simulink model "Flexible_Beam_LP_Simple"  (R2014a)
settings: Solver=ode23t  StartTime=0.0  StopTime=200  RelTol=1e-3  AbsTol=1e-6
PreLoadFcn:
  | Cantilever_Beam_MS2G_Parameters
PostLoadFcn:
  | warning off Simulink:Engine:UsingDefaultMaxStepSize
  | warning off Simulink:Engine:SaveWithParameterizedLinks_Warning
undefined symbols (not defined in the file or in its folder): beam_wall, beam_width, Extr_Data_Box, X, Y, Z
undefined symbols (not defined in the file): beam_length, Damping, density, kbendingx, kbendingy, kelongz, ktwistz, num_elem, shearM, youngsM
libraries: sm_lib x217, nesl_utility x5
(part 1 of 6)
Description:
  | Copyright 2014 The MathWorks, Inc.
settings Model: Creator=smiller  LastModifiedBy=smiller
settings DebuggingCC: UnderspecifiedInitializationDetection=Classic  StateNameClashWarn=warning
settings ExplorerConfigSet: InternalSimMechanicsExplorerSettings="<ExplorerConfiguration><canonicalview>default</canonicalview><AnimationSetting><BasePlaybackSpeed>1.0</BasePlaybackSpeed><PlaybackSpeedFactor>1.0</PlaybackSpeedFactor></AnimationSetting><TilePanel><TileInfo><Tiles Columns=\"1\" Count=\"1\" Rows=\"1\"><Column Left=\"2\" Weight=\"1\"/><Column Left=\"626\"/><Row Top=\"2\" Weight=\"1\"/><Row Top=\"393\"/><Tile Height=\"1\" Width=\"1\" X=\"0\" Y=\"0\"/></Tiles></TileInfo><SceneInfo><SceneViewer><BGColor><R>0.60000002384185791</R><G>0.60000002384185791</G><B>0.60000002384185791</B></BGColor><Camera><Position><X>46.577974053951756</X><Y>-0.39590861008534267</Y><Z>0.29453050072829112</Z></Position><Center><X>15.001379163844208</X><Y>-0.52106864873913594</Y><Z>0.1428630073847893</Z></Center><Up><X>-0.0040091656961971532</X><Y>0.99994673738277207</Y><Z>0.0095104672845314226</Z></Up><Left>-1.0637916226228141</Left><Right>1.0637916226228141</Right><Bottom>-1.031964585942253</Bottom><Top>1.031964585942253</Top></Camera></SceneViewer></SceneInfo></TilePanel></ExplorerConfiguration>"

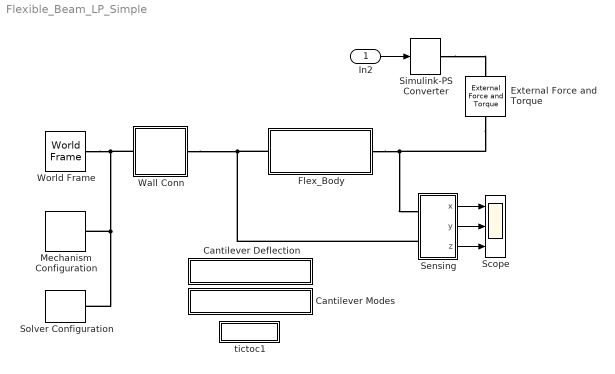
== system Flexible_Beam_LP_Simple ==
  In2 : Inport
  Cantilever Deflection : Subsystem
      settings: OpenFcn=|
      | mdl = bdroot;
      | 
      | load_system('FlexBeamElement_MS2G_Lib')
      | set_param('FlexBeamElement_MS2G_Lib', 'Lock', 'off');
      | set_param('FlexBeamElement_MS2G_Lib/Flex_Element','BlockChoice','Full')
      | 
      | open_system(mdl);
      | open_system([mdl, '/Scope']);
      | set_param([bdroot '/Wall Conn'],'OverrideUsingVariant','Fixed');
      | %set_param([mdl, '/Sensing/Transform Sensor'],'MeasurementFrame','World')
      | 
      | sim(mdl);
      | disp(['Static Deflection is ' num2str(TipDef.signals(2).values(end)) ' m'])
      mask Display: disp('Cantilever Deflection');
  Cantilever Modes : Subsystem
      settings: OpenFcn=Cantilever_Modes_Shapes_MS2G
      mask Display: disp('Cantilever Modes');
  External Force and Torque : sm_lib/Forces and Torques/External Force and Torque  ForceResolutionFrame=AttachedFrame  EnableForceX=off  EnableForceY=on  EnableForceZ=off  EnableForce=off  TorqueResolutionFrame=AttachedFrame  EnableTorqueX=off  EnableTorqueY=off  EnableTorqueZ=off  EnableTorque=off  BlockFunction=simmechanics.library.forces_torques.external_force_torque
  Flex_Body : Subsystem  mask(Flexible Body){rho=density, youngsM=youngsM, shearM=shearM, numelem=num_elem, beam_length=beam_length, beam_width=beam_width, beam_wall=beam_wall, b=Damping}
      mask prompts: rho "Material Density (kg/(m^3)"; youngsM "Modulus of Elasticity (N/m2)"; shearM "Shear Modulus (N/m2)"; numelem "Number of elements"; beam_length "Beam Length (m)"; beam_width "Beam Width & Height (m)"; beam_wall "Beam Wall Thickness(m)"; b "Damping Constant (Nm/rad.s)"
      mask help:
      | Models a flexible hollow square beam based on lumped parameter method.
      | Number of flexible elements, material properties as well as beam
      | dimension can be varied from mask parameters.
      mask init:
      | [kbendingx, kbendingy, ktwistz, kelongz, length] = Compute_GFE_Prop(rho, youngsM, shearM, numelem, beam_length, beam_width,beam_wall);
      | thisblock = gcb;
      | anno = ['No of Elem: ' num2str(numelem)];
      | set_param(thisblock, 'AttributesFormatString',anno);
      | if numelem <1
      |     error('Number of Flexible elements should be greater than 0')
      | end
      | prev_flex_bod = find_system(gcb,'LookUnderMasks','all','RegExp','on','Name','Flex_Elem_*');
      | if ~isempty(prev_flex_bod)
      |     delete_block(prev_flex_bod(1:end))
      | end
      | linehan = find_system(thisblock,'LookUnderMasks','all','FindAll','on','type','line');
      | if ~isempty(linehan)
      |     delete_line(linehan)
      | end
      | blk_or = [100 155 140 195];
      | set_param([thisblock '/B'],'Position',blk_or)
      | set_param([thisblock '/' sprintf('Transform\nBeamX')],'Position',blk_or+[80 0 80 0])
      | add_line(thisblock,['B/Rconn1'],[sprintf('Transform\nBeamX') '/Lconn1'],'autorouting','on');
      | add_block('FlexBeamElement_MS2G_Lib/Bend_Simple',[thisblock '/Flex_Elem_' num2str(1)],'Position',blk_or+[80 0 80 0]*2)
      | add_line(thisblock,[sprintf('Transform\nBeamX') '/Rconn1'],['Flex_Elem_' num2str(1) '/Lconn1'],'autorouting','on');
      | set_param([thisblock '/Flex_Elem_' num2str(1)], 'LinkStatus', 'none')
      | state_order{1} = [thisblock '/Flex_Elem_' num2str(1) '/Revolute Joint'];
      | for i = 2:1:numelem
      |     add_block('FlexBeamElement_MS2G_Lib/Bend_Simple',[thisblock '/Flex_Elem_' num2str(i)],'Position',blk_or+(i+1)*[80 0 80 0])
      |     add_line(thisblock,['Flex_Elem_' num2str(i-1) '/Rconn1'],['Flex_Elem_' num2str(i) '/Lconn1'],'autorouting','on');
      |     set_param([thisblock '/Flex_Elem_' num2str(i)], 'LinkStatus', 'none')
      |     state_order{i} = [thisblock '/Flex_Elem_' num2str(i) '/Revolute Joint'];
      | end
      | set_param([thisblock '/F'],'Position',blk_or+ (numelem+2)*[80 0 80 0]);
      | add_line(thisblock,['Flex_Elem_' num2str(numelem) '/Rconn1'],['F/Rconn1'],'autorouting','on');
      | assignin('base','State_order',state_order)
      settings: AttributesFormatString=No of Elem: 30  CopyFcn=set_param(gcb, 'LinkStatus', 'none')
      mask Display:
      | image(imread('Flexible_Beam.png'));
      | color red
      | port_label('LConn',1,'B');
      | port_label('RConn',1,'F');
  Mechanism Configuration : sm_lib/Utilities/Mechanism Configuration  UniformGravity=Constant  GravityVector=gravity  GravityUnits=m/s^2  LinearizationDelta=0.001  BlockFunction=simmechanics.library.utilities.mechanism_configuration
  Scope : Scope  NumInputPorts=3
      settings: YMin=29.8~-1.5~-0.001  YMax=30.2~0~0.001  SaveName=TipDef
  Sensing : Subsystem
  Simulink-PS Converter : nesl_utility/Simulink-PS Converter  PhysicalDomain=network_engine_domain  SubClassName=ps_input  LeftPortType=input  RightPortType=output  PseudoPeriodic=off  Frequencies=[]  NoiseDistribution=none  NoiseParameters=[]  Unit=1  AffineConversion=off  InputFiltering=off  SimscapeFilterOrder=1  InputFilterTimeConstant=0.001  UdotUserProvided=1
  Solver Configuration : nesl_utility/Solver Configuration  PhysicalDomain=network_engine_domain  SubClassName=solver  LeftPortType=input  RightPortType=generic  Accelerate=off  Tones=[]  Harmonics=[]  SimulateNoise=off  Profile=off  UseLocalSampling=off  EnableSwitchedLinearOptims=on  FrequencyDomain=off  UseCCode=off  RelTol=0.001  AbsTol=1e-06  MinStep=1e-09  ToWorkspace=off  DoDC=off  ResidualTolerance=1e-09  UseLocalSolver=off  LocalSolverChoice=NE_BACKWARD_EULER_ADVANCER  LocalSolverSampleTime=0.001  DoFixedCost=off  MaxNonlinIter=3  MaxModeIter=2  LinearAlgebra=Sparse  DelaysMemoryBudget=1024  AutomaticFiltering=on  FilteringTimeConstant=0.001
  Wall Conn : Subsystem  Variant=on  OverrideUsingVariant=Fixed
      mask Display:
      | if strcmp(get_param(gcb,'ActiveVariant'),'Fixed')
      |     image(imread('Weld_Image.png'))
      | else
      |     image(imread('Rev_Image.png'))
      | end
      | color red
      | port_label('LConn',1,'B');
      | port_label('Rconn',1,'F');
  World Frame : sm_lib/Frames and Transforms/World Frame  BlockFunction=simmechanics.library.frames_transforms.world_frame
  tictoc1 : Subsystem
      settings: OpenFcn=open('Flexible_Beam_Demo_Script.html')
      mask Display: disp('Script')
  wires:
  In2/1 -> Simulink-PS Converter/1
  Sensing/1(x) -> Scope/1
  Sensing/2(y) -> Scope/2
  Sensing/3(z) -> Scope/3
  connections:
  Simulink-PS Converter/RConn1 -- External Force and Torque/LConn1
  External Force and Torque/RConn1 -- Flex_Body/RConn1 -- Sensing/LConn1
  Solver Configuration/RConn1 -- Wall Conn/LConn1 -- World Frame/RConn1 -- Mechanism Configuration/RConn1
  Sensing/LConn2 -- Flex_Body/LConn1 -- Wall Conn/RConn1

== system Flexible_Beam_LP_Simple/Cantilever Deflection ==

== system Flexible_Beam_LP_Simple/Cantilever Modes ==

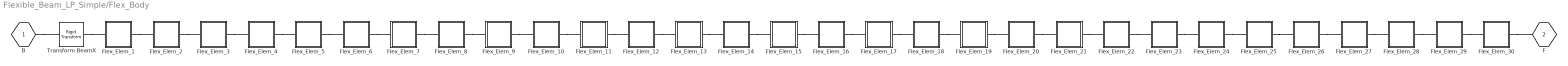
== system Flexible_Beam_LP_Simple/Flex_Body ==
  Flex_Elem_1 : Subsystem  mask{length=length, rho=rho, beam_width=beam_width, beam_wall=beam_wall, kbendingx=kbendingx, kbendingy=kbendingy, kbendingz=ktwistz, kelongz=kelongz, b=b}
      mask prompts: length "Beam Length (m)"; rho "Material Density (kg/(m^3)"; beam_width "Beam Width & Height (m)"; beam_wall "Beam Wall Thickness (m)"; kbendingx "Bending Spring Constant about X(Nm/rad)"; kbendingy "Bending Spring Constant about Y(Nm/rad)"; kbendingz "Twist Spring Constant about Z(Nm/rad)"; kelongz "Elongation Spring Constant about Z(N/m)"; b "Damping Constant (Nm/rad.s)"
  Flex_Elem_10 : Subsystem  mask{length=length, rho=rho, beam_width=beam_width, beam_wall=beam_wall, kbendingx=kbendingx, kbendingy=kbendingy, kbendingz=ktwistz, kelongz=kelongz, b=b}
      mask prompts: length "Beam Length (m)"; rho "Material Density (kg/(m^3)"; beam_width "Beam Width & Height (m)"; beam_wall "Beam Wall Thickness (m)"; kbendingx "Bending Spring Constant about X(Nm/rad)"; kbendingy "Bending Spring Constant about Y(Nm/rad)"; kbendingz "Twist Spring Constant about Z(Nm/rad)"; kelongz "Elongation Spring Constant about Z(N/m)"; b "Damping Constant (Nm/rad.s)"
  Flex_Elem_11 : Subsystem  mask{length=length, rho=rho, beam_width=beam_width, beam_wall=beam_wall, kbendingx=kbendingx, kbendingy=kbendingy, kbendingz=ktwistz, kelongz=kelongz, b=b}
      mask prompts: length "Beam Length (m)"; rho "Material Density (kg/(m^3)"; beam_width "Beam Width & Height (m)"; beam_wall "Beam Wall Thickness (m)"; kbendingx "Bending Spring Constant about X(Nm/rad)"; kbendingy "Bending Spring Constant about Y(Nm/rad)"; kbendingz "Twist Spring Constant about Z(Nm/rad)"; kelongz "Elongation Spring Constant about Z(N/m)"; b "Damping Constant (Nm/rad.s)"
  Flex_Elem_12 : Subsystem  mask{length=length, rho=rho, beam_width=beam_width, beam_wall=beam_wall, kbendingx=kbendingx, kbendingy=kbendingy, kbendingz=ktwistz, kelongz=kelongz, b=b}
      mask prompts: length "Beam Length (m)"; rho "Material Density (kg/(m^3)"; beam_width "Beam Width & Height (m)"; beam_wall "Beam Wall Thickness (m)"; kbendingx "Bending Spring Constant about X(Nm/rad)"; kbendingy "Bending Spring Constant about Y(Nm/rad)"; kbendingz "Twist Spring Constant about Z(Nm/rad)"; kelongz "Elongation Spring Constant about Z(N/m)"; b "Damping Constant (Nm/rad.s)"
  Flex_Elem_13 : Subsystem  mask{length=length, rho=rho, beam_width=beam_width, beam_wall=beam_wall, kbendingx=kbendingx, kbendingy=kbendingy, kbendingz=ktwistz, kelongz=kelongz, b=b}
      mask prompts: length "Beam Length (m)"; rho "Material Density (kg/(m^3)"; beam_width "Beam Width & Height (m)"; beam_wall "Beam Wall Thickness (m)"; kbendingx "Bending Spring Constant about X(Nm/rad)"; kbendingy "Bending Spring Constant about Y(Nm/rad)"; kbendingz "Twist Spring Constant about Z(Nm/rad)"; kelongz "Elongation Spring Constant about Z(N/m)"; b "Damping Constant (Nm/rad.s)"
  Flex_Elem_14 : Subsystem  mask{length=length, rho=rho, beam_width=beam_width, beam_wall=beam_wall, kbendingx=kbendingx, kbendingy=kbendingy, kbendingz=ktwistz, kelongz=kelongz, b=b}
      mask prompts: length "Beam Length (m)"; rho "Material Density (kg/(m^3)"; beam_width "Beam Width & Height (m)"; beam_wall "Beam Wall Thickness (m)"; kbendingx "Bending Spring Constant about X(Nm/rad)"; kbendingy "Bending Spring Constant about Y(Nm/rad)"; kbendingz "Twist Spring Constant about Z(Nm/rad)"; kelongz "Elongation Spring Constant about Z(N/m)"; b "Damping Constant (Nm/rad.s)"
  Flex_Elem_15 : Subsystem  mask{length=length, rho=rho, beam_width=beam_width, beam_wall=beam_wall, kbendingx=kbendingx, kbendingy=kbendingy, kbendingz=ktwistz, kelongz=kelongz, b=b}
      mask prompts: length "Beam Length (m)"; rho "Material Density (kg/(m^3)"; beam_width "Beam Width & Height (m)"; beam_wall "Beam Wall Thickness (m)"; kbendingx "Bending Spring Constant about X(Nm/rad)"; kbendingy "Bending Spring Constant about Y(Nm/rad)"; kbendingz "Twist Spring Constant about Z(Nm/rad)"; kelongz "Elongation Spring Constant about Z(N/m)"; b "Damping Constant (Nm/rad.s)"
  Flex_Elem_16 : Subsystem  mask{length=length, rho=rho, beam_width=beam_width, beam_wall=beam_wall, kbendingx=kbendingx, kbendingy=kbendingy, kbendingz=ktwistz, kelongz=kelongz, b=b}
      mask prompts: length "Beam Length (m)"; rho "Material Density (kg/(m^3)"; beam_width "Beam Width & Height (m)"; beam_wall "Beam Wall Thickness (m)"; kbendingx "Bending Spring Constant about X(Nm/rad)"; kbendingy "Bending Spring Constant about Y(Nm/rad)"; kbendingz "Twist Spring Constant about Z(Nm/rad)"; kelongz "Elongation Spring Constant about Z(N/m)"; b "Damping Constant (Nm/rad.s)"
  Flex_Elem_17 : Subsystem  mask{length=length, rho=rho, beam_width=beam_width, beam_wall=beam_wall, kbendingx=kbendingx, kbendingy=kbendingy, kbendingz=ktwistz, kelongz=kelongz, b=b}
      mask prompts: length "Beam Length (m)"; rho "Material Density (kg/(m^3)"; beam_width "Beam Width & Height (m)"; beam_wall "Beam Wall Thickness (m)"; kbendingx "Bending Spring Constant about X(Nm/rad)"; kbendingy "Bending Spring Constant about Y(Nm/rad)"; kbendingz "Twist Spring Constant about Z(Nm/rad)"; kelongz "Elongation Spring Constant about Z(N/m)"; b "Damping Constant (Nm/rad.s)"
  Flex_Elem_18 : Subsystem  mask{length=length, rho=rho, beam_width=beam_width, beam_wall=beam_wall, kbendingx=kbendingx, kbendingy=kbendingy, kbendingz=ktwistz, kelongz=kelongz, b=b}
      mask prompts: length "Beam Length (m)"; rho "Material Density (kg/(m^3)"; beam_width "Beam Width & Height (m)"; beam_wall "Beam Wall Thickness (m)"; kbendingx "Bending Spring Constant about X(Nm/rad)"; kbendingy "Bending Spring Constant about Y(Nm/rad)"; kbendingz "Twist Spring Constant about Z(Nm/rad)"; kelongz "Elongation Spring Constant about Z(N/m)"; b "Damping Constant (Nm/rad.s)"
  Flex_Elem_19 : Subsystem  mask{length=length, rho=rho, beam_width=beam_width, beam_wall=beam_wall, kbendingx=kbendingx, kbendingy=kbendingy, kbendingz=ktwistz, kelongz=kelongz, b=b}
      mask prompts: length "Beam Length (m)"; rho "Material Density (kg/(m^3)"; beam_width "Beam Width & Height (m)"; beam_wall "Beam Wall Thickness (m)"; kbendingx "Bending Spring Constant about X(Nm/rad)"; kbendingy "Bending Spring Constant about Y(Nm/rad)"; kbendingz "Twist Spring Constant about Z(Nm/rad)"; kelongz "Elongation Spring Constant about Z(N/m)"; b "Damping Constant (Nm/rad.s)"
  Flex_Elem_2 : Subsystem  mask{length=length, rho=rho, beam_width=beam_width, beam_wall=beam_wall, kbendingx=kbendingx, kbendingy=kbendingy, kbendingz=ktwistz, kelongz=kelongz, b=b}
      mask prompts: length "Beam Length (m)"; rho "Material Density (kg/(m^3)"; beam_width "Beam Width & Height (m)"; beam_wall "Beam Wall Thickness (m)"; kbendingx "Bending Spring Constant about X(Nm/rad)"; kbendingy "Bending Spring Constant about Y(Nm/rad)"; kbendingz "Twist Spring Constant about Z(Nm/rad)"; kelongz "Elongation Spring Constant about Z(N/m)"; b "Damping Constant (Nm/rad.s)"
  Flex_Elem_20 : Subsystem  mask{length=length, rho=rho, beam_width=beam_width, beam_wall=beam_wall, kbendingx=kbendingx, kbendingy=kbendingy, kbendingz=ktwistz, kelongz=kelongz, b=b}
      mask prompts: length "Beam Length (m)"; rho "Material Density (kg/(m^3)"; beam_width "Beam Width & Height (m)"; beam_wall "Beam Wall Thickness (m)"; kbendingx "Bending Spring Constant about X(Nm/rad)"; kbendingy "Bending Spring Constant about Y(Nm/rad)"; kbendingz "Twist Spring Constant about Z(Nm/rad)"; kelongz "Elongation Spring Constant about Z(N/m)"; b "Damping Constant (Nm/rad.s)"
  Flex_Elem_21 : Subsystem  mask{length=length, rho=rho, beam_width=beam_width, beam_wall=beam_wall, kbendingx=kbendingx, kbendingy=kbendingy, kbendingz=ktwistz, kelongz=kelongz, b=b}
      mask prompts: length "Beam Length (m)"; rho "Material Density (kg/(m^3)"; beam_width "Beam Width & Height (m)"; beam_wall "Beam Wall Thickness (m)"; kbendingx "Bending Spring Constant about X(Nm/rad)"; kbendingy "Bending Spring Constant about Y(Nm/rad)"; kbendingz "Twist Spring Constant about Z(Nm/rad)"; kelongz "Elongation Spring Constant about Z(N/m)"; b "Damping Constant (Nm/rad.s)"
  Flex_Elem_22 : Subsystem  mask{length=length, rho=rho, beam_width=beam_width, beam_wall=beam_wall, kbendingx=kbendingx, kbendingy=kbendingy, kbendingz=ktwistz, kelongz=kelongz, b=b}
      mask prompts: length "Beam Length (m)"; rho "Material Density (kg/(m^3)"; beam_width "Beam Width & Height (m)"; beam_wall "Beam Wall Thickness (m)"; kbendingx "Bending Spring Constant about X(Nm/rad)"; kbendingy "Bending Spring Constant about Y(Nm/rad)"; kbendingz "Twist Spring Constant about Z(Nm/rad)"; kelongz "Elongation Spring Constant about Z(N/m)"; b "Damping Constant (Nm/rad.s)"
  Flex_Elem_23 : Subsystem  mask{length=length, rho=rho, beam_width=beam_width, beam_wall=beam_wall, kbendingx=kbendingx, kbendingy=kbendingy, kbendingz=ktwistz, kelongz=kelongz, b=b}
      mask prompts: length "Beam Length (m)"; rho "Material Density (kg/(m^3)"; beam_width "Beam Width & Height (m)"; beam_wall "Beam Wall Thickness (m)"; kbendingx "Bending Spring Constant about X(Nm/rad)"; kbendingy "Bending Spring Constant about Y(Nm/rad)"; kbendingz "Twist Spring Constant about Z(Nm/rad)"; kelongz "Elongation Spring Constant about Z(N/m)"; b "Damping Constant (Nm/rad.s)"
  Flex_Elem_24 : Subsystem  mask{length=length, rho=rho, beam_width=beam_width, beam_wall=beam_wall, kbendingx=kbendingx, kbendingy=kbendingy, kbendingz=ktwistz, kelongz=kelongz, b=b}
      mask prompts: length "Beam Length (m)"; rho "Material Density (kg/(m^3)"; beam_width "Beam Width & Height (m)"; beam_wall "Beam Wall Thickness (m)"; kbendingx "Bending Spring Constant about X(Nm/rad)"; kbendingy "Bending Spring Constant about Y(Nm/rad)"; kbendingz "Twist Spring Constant about Z(Nm/rad)"; kelongz "Elongation Spring Constant about Z(N/m)"; b "Damping Constant (Nm/rad.s)"
  Flex_Elem_25 : Subsystem  mask{length=length, rho=rho, beam_width=beam_width, beam_wall=beam_wall, kbendingx=kbendingx, kbendingy=kbendingy, kbendingz=ktwistz, kelongz=kelongz, b=b}
      mask prompts: length "Beam Length (m)"; rho "Material Density (kg/(m^3)"; beam_width "Beam Width & Height (m)"; beam_wall "Beam Wall Thickness (m)"; kbendingx "Bending Spring Constant about X(Nm/rad)"; kbendingy "Bending Spring Constant about Y(Nm/rad)"; kbendingz "Twist Spring Constant about Z(Nm/rad)"; kelongz "Elongation Spring Constant about Z(N/m)"; b "Damping Constant (Nm/rad.s)"
  Flex_Elem_26 : Subsystem  mask{length=length, rho=rho, beam_width=beam_width, beam_wall=beam_wall, kbendingx=kbendingx, kbendingy=kbendingy, kbendingz=ktwistz, kelongz=kelongz, b=b}
      mask prompts: length "Beam Length (m)"; rho "Material Density (kg/(m^3)"; beam_width "Beam Width & Height (m)"; beam_wall "Beam Wall Thickness (m)"; kbendingx "Bending Spring Constant about X(Nm/rad)"; kbendingy "Bending Spring Constant about Y(Nm/rad)"; kbendingz "Twist Spring Constant about Z(Nm/rad)"; kelongz "Elongation Spring Constant about Z(N/m)"; b "Damping Constant (Nm/rad.s)"
  Flex_Elem_27 : Subsystem  mask{length=length, rho=rho, beam_width=beam_width, beam_wall=beam_wall, kbendingx=kbendingx, kbendingy=kbendingy, kbendingz=ktwistz, kelongz=kelongz, b=b}
      mask prompts: length "Beam Length (m)"; rho "Material Density (kg/(m^3)"; beam_width "Beam Width & Height (m)"; beam_wall "Beam Wall Thickness (m)"; kbendingx "Bending Spring Constant about X(Nm/rad)"; kbendingy "Bending Spring Constant about Y(Nm/rad)"; kbendingz "Twist Spring Constant about Z(Nm/rad)"; kelongz "Elongation Spring Constant about Z(N/m)"; b "Damping Constant (Nm/rad.s)"
  Flex_Elem_28 : Subsystem  mask{length=length, rho=rho, beam_width=beam_width, beam_wall=beam_wall, kbendingx=kbendingx, kbendingy=kbendingy, kbendingz=ktwistz, kelongz=kelongz, b=b}
      mask prompts: length "Beam Length (m)"; rho "Material Density (kg/(m^3)"; beam_width "Beam Width & Height (m)"; beam_wall "Beam Wall Thickness (m)"; kbendingx "Bending Spring Constant about X(Nm/rad)"; kbendingy "Bending Spring Constant about Y(Nm/rad)"; kbendingz "Twist Spring Constant about Z(Nm/rad)"; kelongz "Elongation Spring Constant about Z(N/m)"; b "Damping Constant (Nm/rad.s)"
  Flex_Elem_29 : Subsystem  mask{length=length, rho=rho, beam_width=beam_width, beam_wall=beam_wall, kbendingx=kbendingx, kbendingy=kbendingy, kbendingz=ktwistz, kelongz=kelongz, b=b}
      mask prompts: length "Beam Length (m)"; rho "Material Density (kg/(m^3)"; beam_width "Beam Width & Height (m)"; beam_wall "Beam Wall Thickness (m)"; kbendingx "Bending Spring Constant about X(Nm/rad)"; kbendingy "Bending Spring Constant about Y(Nm/rad)"; kbendingz "Twist Spring Constant about Z(Nm/rad)"; kelongz "Elongation Spring Constant about Z(N/m)"; b "Damping Constant (Nm/rad.s)"
  Flex_Elem_3 : Subsystem  mask{length=length, rho=rho, beam_width=beam_width, beam_wall=beam_wall, kbendingx=kbendingx, kbendingy=kbendingy, kbendingz=ktwistz, kelongz=kelongz, b=b}
      mask prompts: length "Beam Length (m)"; rho "Material Density (kg/(m^3)"; beam_width "Beam Width & Height (m)"; beam_wall "Beam Wall Thickness (m)"; kbendingx "Bending Spring Constant about X(Nm/rad)"; kbendingy "Bending Spring Constant about Y(Nm/rad)"; kbendingz "Twist Spring Constant about Z(Nm/rad)"; kelongz "Elongation Spring Constant about Z(N/m)"; b "Damping Constant (Nm/rad.s)"
  Flex_Elem_30 : Subsystem  mask{length=length, rho=rho, beam_width=beam_width, beam_wall=beam_wall, kbendingx=kbendingx, kbendingy=kbendingy, kbendingz=ktwistz, kelongz=kelongz, b=b}
      mask prompts: length "Beam Length (m)"; rho "Material Density (kg/(m^3)"; beam_width "Beam Width & Height (m)"; beam_wall "Beam Wall Thickness (m)"; kbendingx "Bending Spring Constant about X(Nm/rad)"; kbendingy "Bending Spring Constant about Y(Nm/rad)"; kbendingz "Twist Spring Constant about Z(Nm/rad)"; kelongz "Elongation Spring Constant about Z(N/m)"; b "Damping Constant (Nm/rad.s)"
  Flex_Elem_4 : Subsystem  mask{length=length, rho=rho, beam_width=beam_width, beam_wall=beam_wall, kbendingx=kbendingx, kbendingy=kbendingy, kbendingz=ktwistz, kelongz=kelongz, b=b}
      mask prompts: length "Beam Length (m)"; rho "Material Density (kg/(m^3)"; beam_width "Beam Width & Height (m)"; beam_wall "Beam Wall Thickness (m)"; kbendingx "Bending Spring Constant about X(Nm/rad)"; kbendingy "Bending Spring Constant about Y(Nm/rad)"; kbendingz "Twist Spring Constant about Z(Nm/rad)"; kelongz "Elongation Spring Constant about Z(N/m)"; b "Damping Constant (Nm/rad.s)"
  Flex_Elem_5 : Subsystem  mask{length=length, rho=rho, beam_width=beam_width, beam_wall=beam_wall, kbendingx=kbendingx, kbendingy=kbendingy, kbendingz=ktwistz, kelongz=kelongz, b=b}
      mask prompts: length "Beam Length (m)"; rho "Material Density (kg/(m^3)"; beam_width "Beam Width & Height (m)"; beam_wall "Beam Wall Thickness (m)"; kbendingx "Bending Spring Constant about X(Nm/rad)"; kbendingy "Bending Spring Constant about Y(Nm/rad)"; kbendingz "Twist Spring Constant about Z(Nm/rad)"; kelongz "Elongation Spring Constant about Z(N/m)"; b "Damping Constant (Nm/rad.s)"
  Flex_Elem_6 : Subsystem  mask{length=length, rho=rho, beam_width=beam_width, beam_wall=beam_wall, kbendingx=kbendingx, kbendingy=kbendingy, kbendingz=ktwistz, kelongz=kelongz, b=b}
      mask prompts: length "Beam Length (m)"; rho "Material Density (kg/(m^3)"; beam_width "Beam Width & Height (m)"; beam_wall "Beam Wall Thickness (m)"; kbendingx "Bending Spring Constant about X(Nm/rad)"; kbendingy "Bending Spring Constant about Y(Nm/rad)"; kbendingz "Twist Spring Constant about Z(Nm/rad)"; kelongz "Elongation Spring Constant about Z(N/m)"; b "Damping Constant (Nm/rad.s)"
  Flex_Elem_7 : Subsystem  mask{length=length, rho=rho, beam_width=beam_width, beam_wall=beam_wall, kbendingx=kbendingx, kbendingy=kbendingy, kbendingz=ktwistz, kelongz=kelongz, b=b}
      mask prompts: length "Beam Length (m)"; rho "Material Density (kg/(m^3)"; beam_width "Beam Width & Height (m)"; beam_wall "Beam Wall Thickness (m)"; kbendingx "Bending Spring Constant about X(Nm/rad)"; kbendingy "Bending Spring Constant about Y(Nm/rad)"; kbendingz "Twist Spring Constant about Z(Nm/rad)"; kelongz "Elongation Spring Constant about Z(N/m)"; b "Damping Constant (Nm/rad.s)"
  Flex_Elem_8 : Subsystem  mask{length=length, rho=rho, beam_width=beam_width, beam_wall=beam_wall, kbendingx=kbendingx, kbendingy=kbendingy, kbendingz=ktwistz, kelongz=kelongz, b=b}
      mask prompts: length "Beam Length (m)"; rho "Material Density (kg/(m^3)"; beam_width "Beam Width & Height (m)"; beam_wall "Beam Wall Thickness (m)"; kbendingx "Bending Spring Constant about X(Nm/rad)"; kbendingy "Bending Spring Constant about Y(Nm/rad)"; kbendingz "Twist Spring Constant about Z(Nm/rad)"; kelongz "Elongation Spring Constant about Z(N/m)"; b "Damping Constant (Nm/rad.s)"
  Flex_Elem_9 : Subsystem  mask{length=length, rho=rho, beam_width=beam_width, beam_wall=beam_wall, kbendingx=kbendingx, kbendingy=kbendingy, kbendingz=ktwistz, kelongz=kelongz, b=b}
      mask prompts: length "Beam Length (m)"; rho "Material Density (kg/(m^3)"; beam_width "Beam Width & Height (m)"; beam_wall "Beam Wall Thickness (m)"; kbendingx "Bending Spring Constant about X(Nm/rad)"; kbendingy "Bending Spring Constant about Y(Nm/rad)"; kbendingz "Twist Spring Constant about Z(Nm/rad)"; kelongz "Elongation Spring Constant about Z(N/m)"; b "Damping Constant (Nm/rad.s)"
  Transform BeamX : sm_lib/Frames and Transforms/Rigid Transform  TranslationMethod=StandardAxis  TranslationLengthUnit=m  TranslationStandardAxis=+Z  TranslationStandardOffset=0  TranslationCartesianOffset=[0 0 0]  TranslationROffset=0  TranslationROffsetUnits=m  TranslationZOffset=0  TranslationZOffsetUnits=m  TranslationThetaOffset=0  TranslationThetaOffsetUnits=deg  RotationMethod=StandardAxis  RotationAngleUnits=deg  RotationStandardAxis=+Y  RotationAngle=90  RotationArbitraryAxis=[0 0 1]  FollAlignAxisA=+X  BaseAlignAxisA=+Y  FollAlignAxisB=+Y  BaseAlignAxisB=+Z  BlockFunction=simmechanics.library.frames_transforms.rigid_transform
  B : PMIOPort  Port=1  Side=Left
  F : PMIOPort  Port=2  Side=Right
  connections:
  B/RConn1 -- Transform BeamX/LConn1
  Transform BeamX/RConn1 -- Flex_Elem_1/LConn1
  Flex_Elem_1/RConn1 -- Flex_Elem_2/LConn1
  Flex_Elem_2/RConn1 -- Flex_Elem_3/LConn1
  Flex_Elem_3/RConn1 -- Flex_Elem_4/LConn1
  Flex_Elem_4/RConn1 -- Flex_Elem_5/LConn1
  Flex_Elem_5/RConn1 -- Flex_Elem_6/LConn1
  Flex_Elem_6/RConn1 -- Flex_Elem_7/LConn1
  Flex_Elem_7/RConn1 -- Flex_Elem_8/LConn1
  Flex_Elem_8/RConn1 -- Flex_Elem_9/LConn1
  Flex_Elem_9/RConn1 -- Flex_Elem_10/LConn1
  Flex_Elem_10/RConn1 -- Flex_Elem_11/LConn1
  Flex_Elem_11/RConn1 -- Flex_Elem_12/LConn1
  Flex_Elem_12/RConn1 -- Flex_Elem_13/LConn1
  Flex_Elem_13/RConn1 -- Flex_Elem_14/LConn1
  Flex_Elem_14/RConn1 -- Flex_Elem_15/LConn1
  Flex_Elem_15/RConn1 -- Flex_Elem_16/LConn1
  Flex_Elem_16/RConn1 -- Flex_Elem_17/LConn1
  Flex_Elem_17/RConn1 -- Flex_Elem_18/LConn1
  Flex_Elem_18/RConn1 -- Flex_Elem_19/LConn1
  Flex_Elem_19/RConn1 -- Flex_Elem_20/LConn1
  Flex_Elem_20/RConn1 -- Flex_Elem_21/LConn1
  Flex_Elem_21/RConn1 -- Flex_Elem_22/LConn1
  Flex_Elem_22/RConn1 -- Flex_Elem_23/LConn1
  Flex_Elem_23/RConn1 -- Flex_Elem_24/LConn1
  Flex_Elem_24/RConn1 -- Flex_Elem_25/LConn1
  Flex_Elem_25/RConn1 -- Flex_Elem_26/LConn1
  Flex_Elem_26/RConn1 -- Flex_Elem_27/LConn1
  Flex_Elem_27/RConn1 -- Flex_Elem_28/LConn1
  Flex_Elem_28/RConn1 -- Flex_Elem_29/LConn1
  Flex_Elem_29/RConn1 -- Flex_Elem_30/LConn1
  Flex_Elem_30/RConn1 -- F/RConn1

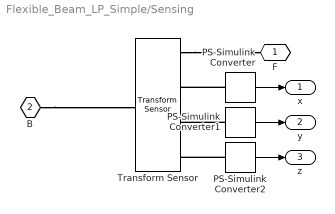
== system Flexible_Beam_LP_Simple/Sensing ==
  PS-Simulink Converter : nesl_utility/PS-Simulink Converter  PhysicalDomain=network_engine_domain  SubClassName=ps_output  LeftPortType=input  RightPortType=output  PseudoPeriodic=off  Frequencies=[]  Unit=1  AffineConversion=off
  PS-Simulink Converter1 : nesl_utility/PS-Simulink Converter  PhysicalDomain=network_engine_domain  SubClassName=ps_output  LeftPortType=input  RightPortType=output  PseudoPeriodic=off  Frequencies=[]  Unit=1  AffineConversion=off
  PS-Simulink Converter2 : nesl_utility/PS-Simulink Converter  PhysicalDomain=network_engine_domain  SubClassName=ps_output  LeftPortType=input  RightPortType=output  PseudoPeriodic=off  Frequencies=[]  Unit=1  AffineConversion=off
  Transform Sensor : sm_lib/Frames and Transforms/Transform Sensor  MeasurementFrame=Base  SenseAngle=off  SenseAxis=off  SenseAngle1=off  SenseAngle2=off  SenseAngle3=off  SenseQ=off  SenseR=off  SenseOmegaX=off  SenseOmegaY=off  SenseOmegaZ=off  SenseOmega1=off  SenseOmega2=off  SenseOmega3=off  SenseQDot=off  SenseRDot=off  SenseAlphaX=off  SenseAlphaY=off  SenseAlphaZ=off  SenseAlpha1=off  SenseAlpha2=off  SenseAlpha3=off  SenseQDDot=off  SenseRDDot=off  SenseX=on  SenseY=on  SenseZ=on  SenseRad=off  SenseAzim=off  SenseDist=off  SenseInc=off  SenseXDot=off  SenseYDot=off  SenseZDot=off  SenseRadDot=off  SenseAzimDot=off  SenseDistDot=off  SenseIncDot=off  SenseXDDot=off  SenseYDDot=off  SenseZDDot=off  SenseRadDDot=off  SenseAzimDDot=off  SenseDistDDot=off  SenseIncDDot=off  BlockFunction=simmechanics.library.frames_transforms.transform_sensor
  F : PMIOPort  Port=1  Side=Left
  B : PMIOPort  Port=2  Side=Left
  x : Outport
  y : Outport  Port=2
  z : Outport  Port=3
  wires:
  PS-Simulink Converter1/1 -> y/1
  PS-Simulink Converter2/1 -> z/1
  PS-Simulink Converter/1 -> x/1
  connections:
  PS-Simulink Converter2/LConn1 -- Transform Sensor/RConn4
  PS-Simulink Converter/LConn1 -- Transform Sensor/RConn2
  PS-Simulink Converter1/LConn1 -- Transform Sensor/RConn3
  B/RConn1 -- Transform Sensor/LConn1
  Transform Sensor/RConn1 -- F/RConn1

== system Flexible_Beam_LP_Simple/Wall Conn ==
  note: 1) Only subsystems can be added as variant choices at this level
      | 2) Blocks cannot be connected at this level as connectivity is
      | automatically determined at simulation, based on the active variant
  Fixed : Subsystem  VariantControl=Fixed
  Rotate : Subsystem  VariantControl=Rotate
  B : PMIOPort  Port=1  Side=Left
  F : PMIOPort  Port=2  Side=Right

== system Flexible_Beam_LP_Simple/tictoc1 ==

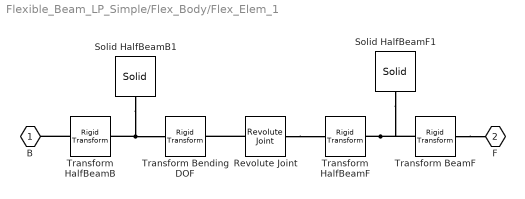
== system Flexible_Beam_LP_Simple/Flex_Body/Flex_Elem_1 ==
  " Transform BeamF" : sm_lib/Frames and Transforms/Rigid Transform  TranslationMethod=StandardAxis  TranslationLengthUnit=m  TranslationStandardAxis=+Z  TranslationStandardOffset=length/4  TranslationCartesianOffset=[0 0 0]  TranslationROffset=0  TranslationROffsetUnits=m  TranslationZOffset=0  TranslationZOffsetUnits=m  TranslationThetaOffset=0  TranslationThetaOffsetUnits=deg  RotationMethod=None  RotationAngleUnits=deg  RotationStandardAxis=+Z  RotationAngle=0  RotationArbitraryAxis=[0 0 1]  FollAlignAxisA=+X  BaseAlignAxisA=+Y  FollAlignAxisB=+Y  BaseAlignAxisB=+Z  BlockFunction=simmechanics.library.frames_transforms.rigid_transform
  " Transform Bending DOF" : sm_lib/Frames and Transforms/Rigid Transform  TranslationMethod=StandardAxis  TranslationLengthUnit=m  TranslationStandardAxis=+Z  TranslationStandardOffset=length/4  TranslationCartesianOffset=[0 0 0]  TranslationROffset=0  TranslationROffsetUnits=m  TranslationZOffset=0  TranslationZOffsetUnits=m  TranslationThetaOffset=0  TranslationThetaOffsetUnits=deg  RotationMethod=StandardAxis  RotationAngleUnits=deg  RotationStandardAxis=+Y  RotationAngle=90  RotationArbitraryAxis=[0 0 1]  FollAlignAxisA=+X  BaseAlignAxisA=+Y  FollAlignAxisB=+Y  BaseAlignAxisB=+Z  BlockFunction=simmechanics.library.frames_transforms.rigid_transform
  Revolute Joint : sm_lib/Joints/Revolute Joint  SenseConstraintForce=off  SenseConstraintForceX=off  SenseConstraintForceY=off  SenseConstraintForceZ=off  SenseConstraintTorque=off  SenseConstraintTorqueX=off  SenseConstraintTorqueY=off  SenseConstraintTorqueZ=off  SenseTotalForce=off  SenseTotalForceX=off  SenseTotalForceY=off  SenseTotalForceZ=off  SenseTotalTorque=off  SenseTotalTorqueX=off  SenseTotalTorqueY=off  SenseTotalTorqueZ=off  CompositeWrenchDir=FollowerOnBase  CompositeWrenchFrame=BaseFrame  EquilibriumPosition=0  EquilibriumPositionUnits=deg  SpringStiffness=kbendingx  SpringStiffnessUnits=N*m/rad  DampingCoefficient=b  DampingCoefficientUnits=N*m/(rad/s)  TorqueActuationMode=NoTorque  MotionActuationMode=ComputedMotion  SensePosition=off  SenseVelocity=off  SenseAcceleration=off  SenseTorqueForce=off  PositionTargetValue=0  PositionTargetValueUnits=deg  PositionTargetSpecify=off  PositionTargetPriority=High  VelocityTargetValue=0  VelocityTargetValueUnits=deg/s  VelocityTargetSpecify=off  VelocityTargetPriority=High  BlockFunction=simmechanics.library.joints.revolute_joint
  Solid HalfBeamB1 : sm_lib/Body Elements/Solid  InertiaType=CalculateFromGeometry  Mass=1  MassUnits=kg  CenterOfMass=[0 0 0]  CenterOfMassUnits=m  MomentsOfInertia=[1 1 1]  MomentsOfInertiaUnits=kg*m^2  ProductsOfInertia=[0 0 0]  ProductsOfInertiaUnits=kg*m^2  DensityBased=on  Density=rho  DensityUnits=kg/(m^3)  GraphicType=FromGeometry  MarkerShape=Sphere  MarkerSize=10  MarkerSizeUnits=m  GraphicVisPropType=SimpleVisualProperties  GraphicDiffuseColor=[0.5 0.5 0.5]  GraphicSpecularColor=[0.5 0.5 0.5 1.0]  GraphicAmbientColor=[0.15 0.15 0.15 1.0]  GraphicEmissiveColor=[0.0 0.0 0.0 1.0]  GraphicShininess=75  GraphicOpacity=1.0  GeometryShape=GeneralExtrusion  RectangleSize=[1 1]  RectangleSizeUnits=m  BrickDimensions=[1 1 1]  BrickDimensionUnits=m  CylinderRadius=1  CylinderRadiusUnits=m  CylinderLength=1  CylinderLengthUnits=m  SphereRadius=1  SphereRadiusUnits=m  EllipsoidRadii=[1 1 1]  EllipsoidRadiiUnits=m  ExtrusionCrossSection=Extr_Data_Box(beam_width,beam_width-2*beam_wall,beam_width,beam_width-2*beam_wall)  ExtrusionCrossSectionUnits=m  ExtrusionLength=length/2  ExtrusionLengthUnits=m  PolygonNumSides=3  PolygonOuterRadius=1  PolygonOuterRadiusUnits=m  ExtGeomFileType=STL  ExtGeomFileUnits=m  RevolutionCrossSection=[1 1; 1 -1; 2 -1; 2 1]  RevolutionCrossSectionUnits=m  RevolutionExtent=Full  RevolutionAngle=180  RevolutionAngleUnits=deg  BlockFunction=simmechanics.library.body_elements.solid
  Solid HalfBeamF1 : sm_lib/Body Elements/Solid  InertiaType=CalculateFromGeometry  Mass=1  MassUnits=kg  CenterOfMass=[0 0 0]  CenterOfMassUnits=m  MomentsOfInertia=[1 1 1]  MomentsOfInertiaUnits=kg*m^2  ProductsOfInertia=[0 0 0]  ProductsOfInertiaUnits=kg*m^2  DensityBased=on  Density=rho  DensityUnits=kg/(m^3)  GraphicType=FromGeometry  MarkerShape=Sphere  MarkerSize=10  MarkerSizeUnits=m  GraphicVisPropType=SimpleVisualProperties  GraphicDiffuseColor=[0.5 0.5 0.5]  GraphicSpecularColor=[0.5 0.5 0.5 1.0]  GraphicAmbientColor=[0.15 0.15 0.15 1.0]  GraphicEmissiveColor=[0.0 0.0 0.0 1.0]  GraphicShininess=75  GraphicOpacity=1.0  GeometryShape=GeneralExtrusion  RectangleSize=[1 1]  RectangleSizeUnits=m  BrickDimensions=[1 1 1]  BrickDimensionUnits=m  CylinderRadius=1  CylinderRadiusUnits=m  CylinderLength=1  CylinderLengthUnits=m  SphereRadius=1  SphereRadiusUnits=m  EllipsoidRadii=[1 1 1]  EllipsoidRadiiUnits=m  ExtrusionCrossSection=Extr_Data_Box(beam_width,beam_width-2*beam_wall,beam_width,beam_width-2*beam_wall)  ExtrusionCrossSectionUnits=m  ExtrusionLength=length/2  ExtrusionLengthUnits=m  PolygonNumSides=3  PolygonOuterRadius=1  PolygonOuterRadiusUnits=m  ExtGeomFileType=STL  ExtGeomFileUnits=m  RevolutionCrossSection=[1 1; 1 -1; 2 -1; 2 1]  RevolutionCrossSectionUnits=m  RevolutionExtent=Full  RevolutionAngle=180  RevolutionAngleUnits=deg  BlockFunction=simmechanics.library.body_elements.solid
  Transform HalfBeamB : sm_lib/Frames and Transforms/Rigid Transform  TranslationMethod=StandardAxis  TranslationLengthUnit=m  TranslationStandardAxis=+Z  TranslationStandardOffset=length/4  TranslationCartesianOffset=[0 0 0]  TranslationROffset=0  TranslationROffsetUnits=m  TranslationZOffset=0  TranslationZOffsetUnits=m  TranslationThetaOffset=0  TranslationThetaOffsetUnits=deg  RotationMethod=None  RotationAngleUnits=deg  RotationStandardAxis=+Z  RotationAngle=0  RotationArbitraryAxis=[0 0 1]  FollAlignAxisA=+X  BaseAlignAxisA=+Y  FollAlignAxisB=+Y  BaseAlignAxisB=+Z  BlockFunction=simmechanics.library.frames_transforms.rigid_transform
  Transform HalfBeamF : sm_lib/Frames and Transforms/Rigid Transform  TranslationMethod=StandardAxis  TranslationLengthUnit=m  TranslationStandardAxis=+Z  TranslationStandardOffset=-length/4  TranslationCartesianOffset=[0 0 0]  TranslationROffset=0  TranslationROffsetUnits=m  TranslationZOffset=0  TranslationZOffsetUnits=m  TranslationThetaOffset=0  TranslationThetaOffsetUnits=deg  RotationMethod=StandardAxis  RotationAngleUnits=deg  RotationStandardAxis=+Y  RotationAngle=90  RotationArbitraryAxis=[0 0 1]  FollAlignAxisA=+X  BaseAlignAxisA=+Y  FollAlignAxisB=+Y  BaseAlignAxisB=+Z  BlockFunction=simmechanics.library.frames_transforms.rigid_transform
  B : PMIOPort  Port=1  Side=Left
  F : PMIOPort  Port=2  Side=Right
  connections:
  " Transform BeamF"/RConn1 -- F/RConn1
  Transform HalfBeamB/LConn1 -- B/RConn1
  Transform HalfBeamF/LConn1 -- " Transform BeamF"/LConn1 -- Solid HalfBeamF1/RConn1
  Solid HalfBeamB1/RConn1 -- Transform HalfBeamB/RConn1 -- " Transform Bending DOF"/LConn1
  Revolute Joint/RConn1 -- Transform HalfBeamF/RConn1
  Revolute Joint/LConn1 -- " Transform Bending DOF"/RConn1

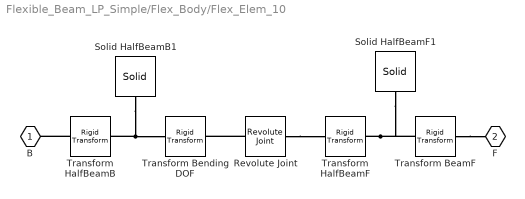
== system Flexible_Beam_LP_Simple/Flex_Body/Flex_Elem_10 ==
  " Transform BeamF" : sm_lib/Frames and Transforms/Rigid Transform  TranslationMethod=StandardAxis  TranslationLengthUnit=m  TranslationStandardAxis=+Z  TranslationStandardOffset=length/4  TranslationCartesianOffset=[0 0 0]  TranslationROffset=0  TranslationROffsetUnits=m  TranslationZOffset=0  TranslationZOffsetUnits=m  TranslationThetaOffset=0  TranslationThetaOffsetUnits=deg  RotationMethod=None  RotationAngleUnits=deg  RotationStandardAxis=+Z  RotationAngle=0  RotationArbitraryAxis=[0 0 1]  FollAlignAxisA=+X  BaseAlignAxisA=+Y  FollAlignAxisB=+Y  BaseAlignAxisB=+Z  BlockFunction=simmechanics.library.frames_transforms.rigid_transform
  " Transform Bending DOF" : sm_lib/Frames and Transforms/Rigid Transform  TranslationMethod=StandardAxis  TranslationLengthUnit=m  TranslationStandardAxis=+Z  TranslationStandardOffset=length/4  TranslationCartesianOffset=[0 0 0]  TranslationROffset=0  TranslationROffsetUnits=m  TranslationZOffset=0  TranslationZOffsetUnits=m  TranslationThetaOffset=0  TranslationThetaOffsetUnits=deg  RotationMethod=StandardAxis  RotationAngleUnits=deg  RotationStandardAxis=+Y  RotationAngle=90  RotationArbitraryAxis=[0 0 1]  FollAlignAxisA=+X  BaseAlignAxisA=+Y  FollAlignAxisB=+Y  BaseAlignAxisB=+Z  BlockFunction=simmechanics.library.frames_transforms.rigid_transform
  Revolute Joint : sm_lib/Joints/Revolute Joint  SenseConstraintForce=off  SenseConstraintForceX=off  SenseConstraintForceY=off  SenseConstraintForceZ=off  SenseConstraintTorque=off  SenseConstraintTorqueX=off  SenseConstraintTorqueY=off  SenseConstraintTorqueZ=off  SenseTotalForce=off  SenseTotalForceX=off  SenseTotalForceY=off  SenseTotalForceZ=off  SenseTotalTorque=off  SenseTotalTorqueX=off  SenseTotalTorqueY=off  SenseTotalTorqueZ=off  CompositeWrenchDir=FollowerOnBase  CompositeWrenchFrame=BaseFrame  EquilibriumPosition=0  EquilibriumPositionUnits=deg  SpringStiffness=kbendingx  SpringStiffnessUnits=N*m/rad  DampingCoefficient=b  DampingCoefficientUnits=N*m/(rad/s)  TorqueActuationMode=NoTorque  MotionActuationMode=ComputedMotion  SensePosition=off  SenseVelocity=off  SenseAcceleration=off  SenseTorqueForce=off  PositionTargetValue=0  PositionTargetValueUnits=deg  PositionTargetSpecify=off  PositionTargetPriority=High  VelocityTargetValue=0  VelocityTargetValueUnits=deg/s  VelocityTargetSpecify=off  VelocityTargetPriority=High  BlockFunction=simmechanics.library.joints.revolute_joint
  Solid HalfBeamB1 : sm_lib/Body Elements/Solid  InertiaType=CalculateFromGeometry  Mass=1  MassUnits=kg  CenterOfMass=[0 0 0]  CenterOfMassUnits=m  MomentsOfInertia=[1 1 1]  MomentsOfInertiaUnits=kg*m^2  ProductsOfInertia=[0 0 0]  ProductsOfInertiaUnits=kg*m^2  DensityBased=on  Density=rho  DensityUnits=kg/(m^3)  GraphicType=FromGeometry  MarkerShape=Sphere  MarkerSize=10  MarkerSizeUnits=m  GraphicVisPropType=SimpleVisualProperties  GraphicDiffuseColor=[0.5 0.5 0.5]  GraphicSpecularColor=[0.5 0.5 0.5 1.0]  GraphicAmbientColor=[0.15 0.15 0.15 1.0]  GraphicEmissiveColor=[0.0 0.0 0.0 1.0]  GraphicShininess=75  GraphicOpacity=1.0  GeometryShape=GeneralExtrusion  RectangleSize=[1 1]  RectangleSizeUnits=m  BrickDimensions=[1 1 1]  BrickDimensionUnits=m  CylinderRadius=1  CylinderRadiusUnits=m  CylinderLength=1  CylinderLengthUnits=m  SphereRadius=1  SphereRadiusUnits=m  EllipsoidRadii=[1 1 1]  EllipsoidRadiiUnits=m  ExtrusionCrossSection=Extr_Data_Box(beam_width,beam_width-2*beam_wall,beam_width,beam_width-2*beam_wall)  ExtrusionCrossSectionUnits=m  ExtrusionLength=length/2  ExtrusionLengthUnits=m  PolygonNumSides=3  PolygonOuterRadius=1  PolygonOuterRadiusUnits=m  ExtGeomFileType=STL  ExtGeomFileUnits=m  RevolutionCrossSection=[1 1; 1 -1; 2 -1; 2 1]  RevolutionCrossSectionUnits=m  RevolutionExtent=Full  RevolutionAngle=180  RevolutionAngleUnits=deg  BlockFunction=simmechanics.library.body_elements.solid
  Solid HalfBeamF1 : sm_lib/Body Elements/Solid  InertiaType=CalculateFromGeometry  Mass=1  MassUnits=kg  CenterOfMass=[0 0 0]  CenterOfMassUnits=m  MomentsOfInertia=[1 1 1]  MomentsOfInertiaUnits=kg*m^2  ProductsOfInertia=[0 0 0]  ProductsOfInertiaUnits=kg*m^2  DensityBased=on  Density=rho  DensityUnits=kg/(m^3)  GraphicType=FromGeometry  MarkerShape=Sphere  MarkerSize=10  MarkerSizeUnits=m  GraphicVisPropType=SimpleVisualProperties  GraphicDiffuseColor=[0.5 0.5 0.5]  GraphicSpecularColor=[0.5 0.5 0.5 1.0]  GraphicAmbientColor=[0.15 0.15 0.15 1.0]  GraphicEmissiveColor=[0.0 0.0 0.0 1.0]  GraphicShininess=75  GraphicOpacity=1.0  GeometryShape=GeneralExtrusion  RectangleSize=[1 1]  RectangleSizeUnits=m  BrickDimensions=[1 1 1]  BrickDimensionUnits=m  CylinderRadius=1  CylinderRadiusUnits=m  CylinderLength=1  CylinderLengthUnits=m  SphereRadius=1  SphereRadiusUnits=m  EllipsoidRadii=[1 1 1]  EllipsoidRadiiUnits=m  ExtrusionCrossSection=Extr_Data_Box(beam_width,beam_width-2*beam_wall,beam_width,beam_width-2*beam_wall)  ExtrusionCrossSectionUnits=m  ExtrusionLength=length/2  ExtrusionLengthUnits=m  PolygonNumSides=3  PolygonOuterRadius=1  PolygonOuterRadiusUnits=m  ExtGeomFileType=STL  ExtGeomFileUnits=m  RevolutionCrossSection=[1 1; 1 -1; 2 -1; 2 1]  RevolutionCrossSectionUnits=m  RevolutionExtent=Full  RevolutionAngle=180  RevolutionAngleUnits=deg  BlockFunction=simmechanics.library.body_elements.solid
  Transform HalfBeamB : sm_lib/Frames and Transforms/Rigid Transform  TranslationMethod=StandardAxis  TranslationLengthUnit=m  TranslationStandardAxis=+Z  TranslationStandardOffset=length/4  TranslationCartesianOffset=[0 0 0]  TranslationROffset=0  TranslationROffsetUnits=m  TranslationZOffset=0  TranslationZOffsetUnits=m  TranslationThetaOffset=0  TranslationThetaOffsetUnits=deg  RotationMethod=None  RotationAngleUnits=deg  RotationStandardAxis=+Z  RotationAngle=0  RotationArbitraryAxis=[0 0 1]  FollAlignAxisA=+X  BaseAlignAxisA=+Y  FollAlignAxisB=+Y  BaseAlignAxisB=+Z  BlockFunction=simmechanics.library.frames_transforms.rigid_transform
  Transform HalfBeamF : sm_lib/Frames and Transforms/Rigid Transform  TranslationMethod=StandardAxis  TranslationLengthUnit=m  TranslationStandardAxis=+Z  TranslationStandardOffset=-length/4  TranslationCartesianOffset=[0 0 0]  TranslationROffset=0  TranslationROffsetUnits=m  TranslationZOffset=0  TranslationZOffsetUnits=m  TranslationThetaOffset=0  TranslationThetaOffsetUnits=deg  RotationMethod=StandardAxis  RotationAngleUnits=deg  RotationStandardAxis=+Y  RotationAngle=90  RotationArbitraryAxis=[0 0 1]  FollAlignAxisA=+X  BaseAlignAxisA=+Y  FollAlignAxisB=+Y  BaseAlignAxisB=+Z  BlockFunction=simmechanics.library.frames_transforms.rigid_transform
  B : PMIOPort  Port=1  Side=Left
  F : PMIOPort  Port=2  Side=Right
  connections:
  " Transform BeamF"/RConn1 -- F/RConn1
  Transform HalfBeamB/LConn1 -- B/RConn1
  Transform HalfBeamF/LConn1 -- " Transform BeamF"/LConn1 -- Solid HalfBeamF1/RConn1
  Solid HalfBeamB1/RConn1 -- Transform HalfBeamB/RConn1 -- " Transform Bending DOF"/LConn1
  Revolute Joint/RConn1 -- Transform HalfBeamF/RConn1
  Revolute Joint/LConn1 -- " Transform Bending DOF"/RConn1
